simulink model "mreuse_basic9"  (Simulink 6.3)
settings: Solver=FixedStepDiscrete  StartTime=0.0  StopTime=10.0  RelTol=1e-3
PreLoadFcn:
  | inlined_m = 3;auto_k = 2;exported_n = 4;
libraries: simulink x1
settings Model: CovMetricSettings=d  Creator=rajbabu  LastModifiedBy=mshakeri  ExtModeEnableOpenProtocolUploading=on  ExtModeOpenProtocolUploadingEqualLengthVectors=off  ExtModeAutoUpdateStatusClock=off  TunableVars=auto_k,exported_n  TunableVarsStorageClass=Auto,ExportedGlobal  TunableVarsTypeQualifier=,  StrictBusMsg=ErrorLevel1
settings OptimizationCC: BlockReduction=off  BooleanDataType=off  InlineParams=on  InlineInvariantSignals=on
settings DebuggingCC: SignalResolutionControl=UseLocalSettings  SolverPrmCheckMsg=none
settings HardwareCC: TargetUnknown=on
settings RTWCC: RetainRTWFile=on

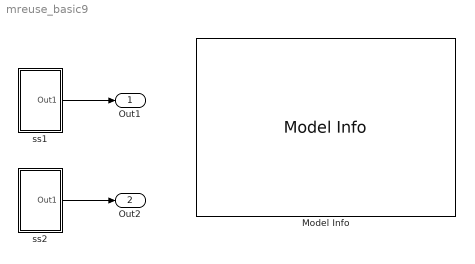
== system mreuse_basic9 ==
  Model Info : simulink/Model-Wide Utilities/Model Info  InitialSaveTempField=mthomas#|#2002/02/26 22:07:01#|#1.8#|#//src/CVS/devel/matlab/test/toolbox/simulink/code_reuse/mreuse_basic9.mdl,v 1.8 2002/02/26 22:07:01 mthomas Exp#|#mreuse_basic9.mdl,v 1.8 2002/02/26 22:07:01 mthomas Exp#|##|#mreuse_basic9.mdl,v#|#//src/CVS/devel/matlab/test/toolbox/simulink/code_reuse/mreuse_basic9.mdl,v#|#Exp#|#  InitialBlockCM=rcs  BlockCM=rcs  Frame=on  SaveTempField=mthomas#|#2002/02/26 22:07:01#|#1.8#|#//src/CVS/devel/matlab/test/toolbox/simulink/code_reuse/mreuse_basic9.mdl,v 1.8 2002/02/26 22:07:01 mthomas Exp#|#mreuse_basic9.mdl,v 1.8 2002/02/26 22:07:01 mthomas Exp#|##|#mreuse_basic9.mdl,v#|#//src/CVS/devel/matlab/test/toolbox/simulink/code_reuse/mreuse_basic9.mdl,v#|#Exp#|#  DisplayStringWithTags=|  HorizontalTextAlignment=Left  LeftAlignmentValue=0.02  SourceBlockDiagram=mreuse_basic9  TagMaxNumber=20  CMTag1=$Author: batserve $  CMTag2=$Date: 2005/06/27 16:30:50 $  CMTag3=$Revision: 1.1.4.1 $  CMTag4=$Header: //src/CVS/devel/matlab/test/toolbox/simulink/modelref/ss2mdlref/Attic/mreuse_basic9.mdl,v 1.1.4.1 2005/06/27 16:30:50 batserve Exp $  CMTag5=$Id: mreuse_basic9.mdl,v 1.1.4.1 2005/06/27 16:30:50 batserve Exp $  CMTag6="$Locker:  $"  CMTag7=$RCSfile: mreuse_basic9.mdl,v $  CMTag8=$Source: //src/CVS/devel/matlab/test/toolbox/simulink/modelref/ss2mdlref/Attic/mreuse_basic9.mdl,v $  CMTag9=$State: Exp $
      | Model Info:
      |  Inline Parameters: On
      |  ss1 = ss2 (reused)
      |  Parameters:
      |   auto_k - SimulinkAuto
      |   exported_n -  ExportedGlobal
      | Purpose:
      |  Inline Parameters - has rtP 
      | 
      | Prototype:
      |  ss1(&rtB.ss1)
  ss1 : Subsystem  Tag=reused(2)  TreatAsAtomicUnit=on
      settings: AttributesFormatString=Tag = %<Tag>
  ss2 : Subsystem  Tag=reused(2)  TreatAsAtomicUnit=on
      settings: AttributesFormatString=Tag = %<Tag>
  Out1 : Outport
  Out2 : Outport  Port=2
  wires:
  ss1/1(Out1) -> Out1/1
  ss2/1(Out1) -> Out2/1

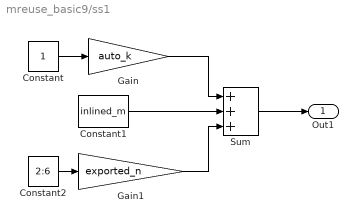
== system mreuse_basic9/ss1 ==
  Constant : Constant
  Constant1 : Constant  Value=inlined_m
  Constant2 : Constant  Value=2:6
  Gain : Gain  Gain=auto_k  SaturateOnIntegerOverflow=on
  Gain1 : Gain  Gain=exported_n  SaturateOnIntegerOverflow=on
  Sum : Sum  Inputs=+++  SaturateOnIntegerOverflow=on  InputSameDT=on
  Out1 : Outport
  wires:
  Constant/1 -> Gain/1
  Gain/1 -> Sum/1
  Sum/1 -> Out1/1
  Constant1/1 -> Sum/2
  Constant2/1 -> Gain1/1
  Gain1/1 -> Sum/3

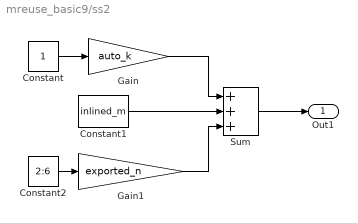
== system mreuse_basic9/ss2 ==
  Constant : Constant
  Constant1 : Constant  Value=inlined_m
  Constant2 : Constant  Value=2:6
  Gain : Gain  Gain=auto_k  SaturateOnIntegerOverflow=on
  Gain1 : Gain  Gain=exported_n  SaturateOnIntegerOverflow=on
  Sum : Sum  Inputs=+++  SaturateOnIntegerOverflow=on  InputSameDT=on
  Out1 : Outport
  wires:
  Constant/1 -> Gain/1
  Gain/1 -> Sum/1
  Sum/1 -> Out1/1
  Constant1/1 -> Sum/2
  Constant2/1 -> Gain1/1
  Gain1/1 -> Sum/3
